simulink library "GenericTarget"  (R2020b)
settings: Solver=VariableStepAuto  StartTime=0.0  StopTime=10.0  RelTol=1e-3
undefined symbols (not defined in the file or in its folder): CheckUniqueParameterValue
(part 1 of 2)
settings Model: Creator=damerius  LastModifiedBy=damerius

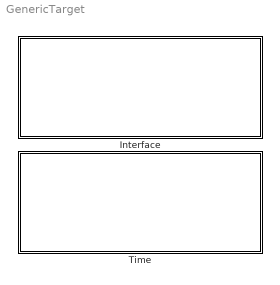
== system GenericTarget ==
  Interface : Subsystem
  Time : Subsystem

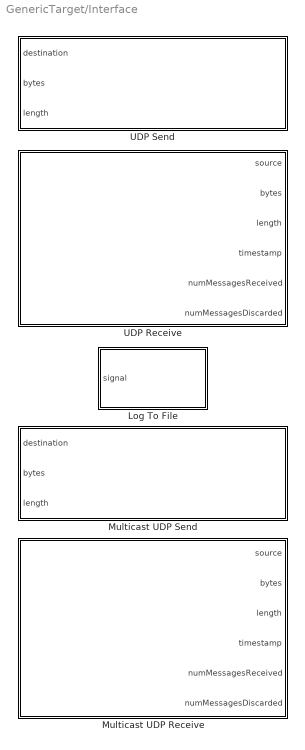
== system GenericTarget/Interface ==
  Log To File : Subsystem  InitFcn=CheckUniqueParameterValue(gcs,gcb,'idLog');  mask{idLog=0, signalDimension=1, labelsLog='label'}
      mask prompts: idLog "Unique ID:"; signalDimension "Signal dimension:"; labelsLog "Signal names, seperated by comma in one string:"
      mask help:
      | Log a signal to a file. This block implements the signal logging functionality on the generic target. During simulation this block has no effect.
      |
      | Internally, the model time is used as timestamp.
      mask DialogControl DescGroupVar Prompt: Log To File - Generic Target
      mask Display:
      | % Get dimension of block
      | pos = get_param(gcb, 'Position');
      | width = pos(3) - pos(1);
      | height = pos(4) - pos(2);
      | 
      | % Set image to center of block
      | imgSize = 32;
      | image('write.svg', [width-imgSize,0.5*(height-imgSize),imgSize,imgSize]);
      | image('icon.svg', [0.5*(width-imgSize),0.5*(height-imgSize),imgSize,imgSize]);
      | 
      | % Show socket port
      | maskStr = get_param(gcb,'idLog');
      | strText = ['ID: ' maskStr];
      | text(0.5*width,0.5*(height-imgSize)-4,strText, 'hor','center','texmode','on');
  Multicast UDP Receive : Subsystem  InitFcn=CheckUniqueParameterValue(gcs,gcb,'interfacePortRX');  mask{interfacePortRX=25000, interfaceIP=[0,0,0,0], groupIP=[239,0,0,0], rxBufferSize=1024, SampleTime=-1, prioritySocket=6, priorityThread=31, ttl=1, maxNumMessages=1, bufferStrategy=Discard oldest message}
      mask prompts: interfacePortRX "Local port:"; interfaceIP "Interface ([0,0,0,0] for default interface):"; groupIP "Group address:"; rxBufferSize "Receive buffer size:"; SampleTime "Sample time (-1 for inherited):"; prioritySocket "Socket priority (0 ... 6, default is 6):"; priorityThread "Receiver thread priority (0 ... 99, default is 31):"; ttl "Time-to-live value associated with multicast traffic for this socket (default is 1)"; maxNumMessages "Maximum number of messages in buffer (default is 1):"; bufferStrategy "Buffer strategy (if buffer is full):"
      mask help:
      | Receive UDP messages from a multicast group. This block implements the UDP multicast receiver functionality on the generic target. If the toolbox was built with the host implementation, then this block behaves similar to the one on the target. Otherwise this block has no effect during simulations.<br><br>
      |
      | <b>source</b><br>A 5-by-M uint16 vector denoting the source address, where M denotes the number of messages in the buffer. The first four values in a column indicate the source IPv4 address (LSB) and the fifth value in a column indicates the source port.<br><br>
      |
      | <b>bytes</b><br>An N-by-M matrix containing the messages that have been received, where N indicates the buffer size for a single message and M denotes the number of messages in the buffer.<br><br>
      |
      | <b>length</b><br>An M-by-1 vector indicating the actual length of the corresponding message.<br><br>
      |
      | <b>timestamp</b><br>An M-by-1 vector indicating the timestamp in seconds (model time) when the corresponding message has been received.<br><br>
      |
      | <b>numMessagesReceived</b><br>The number of messages that have been received.<br><br>
      |
      | <b>numMessagesDiscarded</b><br>The number of messages that have been discarded.
      mask TypeOptions bufferStrategy: Discard oldest message | Discard received message
      mask DialogControl DescGroupVar Prompt: Multicast UDP Receive - Generic Target
      mask DialogControl Container4 Prompt: Parameters
      mask DialogControl Container7 Prompt: Advanced
      mask DialogControl Container6 Prompt: Buffering
      mask Display:
      | % Get dimension of block
      | pos = get_param(gcb, 'Position');
      | width = pos(3) - pos(1);
      | height = pos(4) - pos(2);
      | 
      | % Set image to center of block
      | imgSize = 32;
      | image('rx.svg', [0,0.5*(height-imgSize),imgSize,imgSize]);
      | image('icon.svg', [0.5*(width-imgSize),0.5*(height-imgSize),imgSize,imgSize]);
      | 
      | % Show socket port
      | maskStr = get_param(gcb,'interfacePortRX');
      | strText = ['Port: ' maskStr];
      | text(0.5*width,0.5*(height-imgSize)-4,strText, 'hor','center','texmode','on');
      | 
      | % Show group ip
      | maskStr = get_param(gcb,'groupIP');
      | maskStr = strrep(maskStr,'[','');
      | maskStr = strrep(maskStr,']','');
      | maskStr = strrep(maskStr,',','.');
      | text(0.5*width,0.5*(height+imgSize)+6,maskStr, 'hor','center','texmode','on');
  Multicast UDP Send : Subsystem  mask{interfacePort=25000, groupIP=[239,0,0,0], interfaceIP=[0,0,0,0], SampleTime=-1, prioritySocket=6, priorityThread=31, ttl=1}
      mask prompts: interfacePort "Local port:"; groupIP "Group address:"; interfaceIP "Interface ([0,0,0,0] for default interface):"; SampleTime "Sample time (-1 for inherited):"; prioritySocket "Socket priority (0 ... 6, default is 6):"; priorityThread "Receiver thread priority (0 ... 99, default is 31):"; ttl "Time-to-live value associated with multicast traffic for this socket (default is 1):"
      mask help:
      | Send a UDP message to a specified destination. This block implements the UDP multicast transmission functionality on the generic target. If the toolbox was built with the host implementation, then this block behaves similar to the one on the target. Otherwise this block has no effect during simulations.<br><br>
      |
      | <b>destination</b><br>A 5-by-1 uint16 vector denoting the destination address, where the first four values indicate the destination IPv4 address (LSByte) and the fifth value indicates the destination port.<br><br>
      |
      | <b>bytes</b><br>The message that should be transmitted.<br><br>
      |
      | <b>length</b><br>The number of bytes that should be transmitted.
      mask DialogControl DescGroupVar Prompt: Multicast UDP Send - Generic Target
      mask DialogControl Container4 Prompt: Parameters
      mask DialogControl Container5 Prompt: Advanced
      mask Display:
      | % Get dimension of block
      | pos = get_param(gcb, 'Position');
      | width = pos(3) - pos(1);
      | height = pos(4) - pos(2);
      | 
      | % Set image to center of block
      | imgSize = 32;
      | image('tx.svg', [width-imgSize,0.5*(height-imgSize),imgSize,imgSize]);
      | image('icon.svg', [0.5*(width-imgSize),0.5*(height-imgSize),imgSize,imgSize]);
      | 
      | % Show socket port
      | maskStr = get_param(gcb,'interfacePort');
      | strText = ['Port: ' maskStr];
      | text(0.5*width,0.5*(height-imgSize)-4,strText, 'hor','center','texmode','on');
      | 
      | % Show group ip
      | maskStr = get_param(gcb,'groupIP');
      | maskStr = strrep(maskStr,'[','');
      | maskStr = strrep(maskStr,']','');
      | maskStr = strrep(maskStr,',','.');
      | text(0.5*width,0.5*(height+imgSize)+6,maskStr, 'hor','center','texmode','on');
  UDP Receive : Subsystem  InitFcn=CheckUniqueParameterValue(gcs,gcb,'interfacePortRX');  mask{interfacePortRX=25000, interfaceIP=[0,0,0,0], rxBufferSize=1024, SampleTime=-1, prioritySocket=6, priorityThread=31, maxNumMessages=1, bufferStrategy=Discard oldest message}
      mask prompts: interfacePortRX "Local port:"; interfaceIP "Interface ([0,0,0,0] for default interface):"; rxBufferSize "Receive buffer size:"; SampleTime "Sample time (-1 for inherited):"; prioritySocket "Socket priority (0 ... 6, default is 6):"; priorityThread "Receiver thread priority (0 ... 99, default is 31):"; maxNumMessages "Maximum number of messages in buffer (default is 1):"; bufferStrategy "Buffer strategy (if buffer is full):"
      mask help:
      | Receive UDP messages at the specified port. This block implements the UDP receiver functionality on the generic target. If the toolbox was built with the host implementation, then this block behaves similar to the one on the target. Otherwise this block has no effect during simulations.<br><br>
      |
      | <b>source</b><br>A 5-by-M uint16 vector denoting the source address, where M denotes the number of messages in the buffer. The first four values in a column indicate the source IPv4 address (LSB) and the fifth value in a column indicates the source port.<br><br>
      |
      | <b>bytes</b><br>An N-by-M matrix containing the messages that have been received, where N indicates the buffer size for a single message and M denotes the number of messages in the buffer.<br><br>
      |
      | <b>length</b><br>An M-by-1 vector indicating the actual length of the corresponding message.<br><br>
      |
      | <b>timestamp</b><br>An M-by-1 vector indicating the timestamp in seconds (model time) when the corresponding message has been received.<br><br>
      |
      | <b>numMessagesReceived</b><br>The number of messages that have been received.<br><br>
      |
      | <b>numMessagesDiscarded</b><br>The number of messages that have been discarded.
      mask TypeOptions bufferStrategy: Discard oldest message | Discard received message
      mask DialogControl DescGroupVar Prompt: UDP Receive - Generic Target
      mask DialogControl Container4 Prompt: Parameters
      mask DialogControl Container5 Prompt: Advanced
      mask DialogControl Container8 Prompt: Buffering
      mask Display:
      | % Get dimension of block
      | pos = get_param(gcb, 'Position');
      | width = pos(3) - pos(1);
      | height = pos(4) - pos(2);
      | 
      | % Set image to center of block
      | imgSize = 32;
      | image('rx.svg', [0,0.5*(height-imgSize),imgSize,imgSize]);
      | image('icon.svg', [0.5*(width-imgSize),0.5*(height-imgSize),imgSize,imgSize]);
      | 
      | % Show socket port
      | maskStr = get_param(gcb,'interfacePortRX');
      | strText = ['Port: ' maskStr];
      | text(0.5*width,0.5*(height-imgSize)-4,strText, 'hor','center','texmode','on');
  UDP Send : Subsystem  mask{interfacePort=25000, interfaceIP=[0,0,0,0], SampleTime=-1, prioritySocket=6, priorityThread=31}
      mask prompts: interfacePort "Local port:"; interfaceIP "Interface ([0,0,0,0] for default interface):"; SampleTime "Sample time (-1 for inherited):"; prioritySocket "Socket priority (0 ... 6, default is 6):"; priorityThread "Receiver thread priority (0 ... 99, default is 31):"
      mask help:
      | Send a UDP message to a specified destination. This block implements the UDP transmission functionality on the generic target. If the toolbox was built with the host implementation, then this block behaves similar to the one on the target. Otherwise this block has no effect during simulations.<br><br>
      |
      | <b>destination</b><br>A 5-by-1 uint16 vector denoting the destination address, where the first four values indicate the destination IPv4 address (LSByte) and the fifth value indicates the destination port.<br><br>
      |
      | <b>bytes</b><br>The message that should be transmitted.<br><br>
      |
      | <b>length</b><br>The number of bytes that should be transmitted.
      mask DialogControl DescGroupVar Prompt: UDP Send - Generic Target
      mask DialogControl Container12 Prompt: Parameters
      mask DialogControl Container13 Prompt: Advanced
      mask Display:
      | % Get dimension of block
      | pos = get_param(gcb, 'Position');
      | width = pos(3) - pos(1);
      | height = pos(4) - pos(2);
      | 
      | % Set image to center of block
      | imgSize = 32;
      | image('tx.svg', [width-imgSize,0.5*(height-imgSize),imgSize,imgSize]);
      | image('icon.svg', [0.5*(width-imgSize),0.5*(height-imgSize),imgSize,imgSize]);
      | 
      | % Show socket port
      | maskStr = get_param(gcb,'interfacePort');
      | strText = ['Port: ' maskStr];
      | text(0.5*width,0.5*(height-imgSize)-4,strText, 'hor','center','texmode','on');

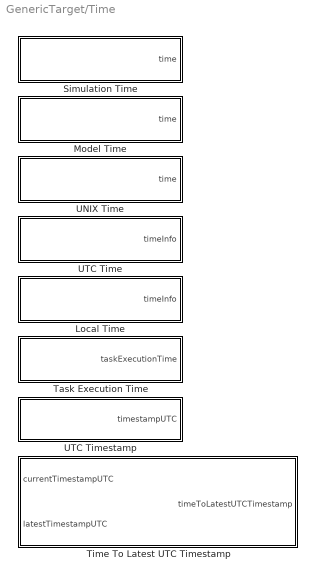
== system GenericTarget/Time ==
  Local Time : Subsystem  mask{SampleTime=-1}
      mask prompts: SampleTime "Sample time (-1 for inherited):"
      mask help:
      | Get the current local time of the target. If the toolbox was not built with the host implementation, then this block has no effect during simulations. If, however, the toolbox was built with the host implementation, then this blocks returns the current local time. The behaviour is different to that one on the target. During simulation each of these blocks returns the local time separately. However, on the target the local time is determined only once per base sampletime.<br><br>
      |
      | <b>nanoseconds</b><br>Nanoseconds after the second [0, 999999999].<br><br>
      |
      | <b>second</b><br>Seconds after the minute [0, 60] (60 to allow leap second).<br><br>
      |
      | <b>minute</b><br>Minutes after the hour [0, 59].<br><br>
      |
      | <b>hour</b><br>Hours since midnight [0, 23].<br><br>
      |
      | <b>mday</b><br>Day of the month [1, 31].<br><br>
      |
      | <b>mon</b><br>Month since January [0, 11].<br><br>
      |
      | <b>year</b><br>Years since 1900.<br><br>
      |
      | <b>wday</b><br>Days since Sunday [0, 6].<br><br>
      |
      | <b>yday</b><br>Days since January 1 [0, 365].<br><br>
      |
      | <b>isdst</b><br>Daylight Saving Time flag. The value is positive if DST is in effect, zero if not and negative if no information is available.
      mask DialogControl DescGroupVar Prompt: Local Time - Generic Target
      mask Display:
      | % Get dimension of block
      | pos = get_param(gcb, 'Position');
      | width = pos(3) - pos(1);
      | height = pos(4) - pos(2);
      | 
      | % Set image to center of block
      | imgSize = 32;
      | image('time.svg', [0.5*(height-imgSize),0.5*(height-imgSize),imgSize,imgSize]);
      | image('icon.svg', [0.5*(width-imgSize),0.5*(height-imgSize),imgSize,imgSize]);
      | 
      | % Set text
      | text(2,2,'Local','horizontalAlignment','left','verticalAlignment','bottom','texmode','on');
  Model Time : Subsystem  mask{SampleTime=-1}
      mask prompts: SampleTime "Sample time (-1 for inherited):"
      mask help:
      | Get the current execution time of the model. If the toolbox was not built with the host implementation, then this block has no effect during simulations. If, however, the toolbox was built with the host implementation, then this blocks returns the measured time to the simulation start. The behaviour is different to that one on the target. During simulation each of these blocks measures the model time separately. However, on the target the model time is measured only once per base sampletime.<br><br>
      |
      | <b>time</b><br>The execution time of the model in seconds.
      mask DialogControl DescGroupVar Prompt: Model Time - Generic Target
      mask Display:
      | % Get dimension of block
      | pos = get_param(gcb, 'Position');
      | width = pos(3) - pos(1);
      | height = pos(4) - pos(2);
      | 
      | % Set image to center of block
      | imgSize = 32;
      | image('time.svg', [0.5*(height-imgSize),0.5*(height-imgSize),imgSize,imgSize]);
      | image('icon.svg', [0.5*(width-imgSize),0.5*(height-imgSize),imgSize,imgSize]);
      | 
      | % Set text
      | text(2,2,'Model','horizontalAlignment','left','verticalAlignment','bottom','texmode','on');
  Simulation Time : Subsystem  mask{SampleTime=-1}
      mask prompts: SampleTime "Sample time (-1 for inherited):"
      mask help:
      | Get the current simulation time of the model. During simulation this block has no effect.<br><br>
      |
      | <b>time</b><br>The simulation time of the model in seconds, that is the number of ticks from of the base rate times the base sample time.
      mask DialogControl DescGroupVar Prompt: Simulation Time - Generic Target
      mask Display:
      | % Get dimension of block
      | pos = get_param(gcb, 'Position');
      | width = pos(3) - pos(1);
      | height = pos(4) - pos(2);
      | 
      | % Set image to center of block
      | imgSize = 32;
      | image('time.svg', [0.5*(height-imgSize),0.5*(height-imgSize),imgSize,imgSize]);
      | image('icon.svg', [0.5*(width-imgSize),0.5*(height-imgSize),imgSize,imgSize]);
      | 
      | % Set text
      | text(2,2,'Simulation','horizontalAlignment','left','verticalAlignment','bottom','texmode','on');
  Task Execution Time : Subsystem  mask{SampleTime=0.001}
      mask prompts: SampleTime "Sample time (<b>must be explicitly specified</b>):"
      mask help: Get the latest task execution time in seconds for the task running at the specified sampletime. During simulation this block has no effect.
      mask DialogControl DescGroupVar Prompt: Task Execution Time - Generic Target
      mask Display:
      | % Get dimension of block
      | pos = get_param(gcb, 'Position');
      | width = pos(3) - pos(1);
      | height = pos(4) - pos(2);
      | 
      | % Set image to center of block
      | imgSize = 32;
      | image('time.svg', [0.5*(height-imgSize),0.5*(height-imgSize),imgSize,imgSize]);
      | image('icon.svg', [0.5*(width-imgSize),0.5*(height-imgSize),imgSize,imgSize]);
      | 
      | % Set text
      | text(2,2,'TET','horizontalAlignment','left','verticalAlignment','bottom','texmode','on');
  Time To Latest UTC Timestamp : Subsystem
      mask help:
      | This block calculates the time difference (seconds) to the latest UTC timestamp. The block only uses standard simulink blocks.<br><br>
      | The basic behaviour is as follows:<br>
      | <b>output</b> = <b>current</b> - <b>latest</b>
      mask DialogControl DescGroupVar Prompt: Time To Latest UTC Timestamp
      mask Display:
      | % Get dimension of block
      | pos = get_param(gcb, 'Position');
      | width = pos(3) - pos(1);
      | height = pos(4) - pos(2);
      | 
      | % Set image to center of block
      | imgSize = 32;
      | image('icon.svg', [0.5*(width-imgSize),0.5*(height-imgSize),imgSize,imgSize]);
  UNIX Time : Subsystem  mask{SampleTime=-1}
      mask prompts: SampleTime "Sample time (-1 for inherited):"
      mask help:
      | Get the current UNIX time. If the toolbox was not built with the host implementation, then this block has no effect during simulations. If, however, the toolbox was built with the host implementation, then this blocks returns the current UNIX time. The behaviour is different to that one on the target. During simulation each of these blocks returns the UNIX time separately. However, on the target the UNIX time is determined only once per base sampletime.<br><br>
      |
      | <b>time</b><br>The UNIX time in seconds. The resolution is one millisecond.
      mask DialogControl DescGroupVar Prompt: UNIX Time - Generic Target
      mask Display:
      | % Get dimension of block
      | pos = get_param(gcb, 'Position');
      | width = pos(3) - pos(1);
      | height = pos(4) - pos(2);
      | 
      | % Set image to center of block
      | imgSize = 32;
      | image('time.svg', [0.5*(height-imgSize),0.5*(height-imgSize),imgSize,imgSize]);
      | image('icon.svg', [0.5*(width-imgSize),0.5*(height-imgSize),imgSize,imgSize]);
      | 
      | % Set text
      | text(2,2,'UNIX','horizontalAlignment','left','verticalAlignment','bottom','texmode','on');
  UTC Time : Subsystem  mask{SampleTime=-1}
      mask prompts: SampleTime "Sample time (-1 for inherited):"
      mask help:
      | Get the current UTC time of the target. If the toolbox was not built with the host implementation, then this block has no effect during simulations. If, however, the toolbox was built with the host implementation, then this blocks returns the current UTC time. The behaviour is different to that one on the target. During simulation each of these blocks returns the UTC time separately. However, on the target the UTC time is determined only once per base sampletime.<br><br>
      |
      | <b>nanoseconds</b><br>Nanoseconds after the second [0, 999999999].<br><br>
      |
      | <b>second</b><br>Seconds after the minute [0, 60] (60 to allow leap second).<br><br>
      |
      | <b>minute</b><br>Minutes after the hour [0, 59].<br><br>
      |
      | <b>hour</b><br>Hours since midnight [0, 23].<br><br>
      |
      | <b>mday</b><br>Day of the month [1, 31].<br><br>
      |
      | <b>mon</b><br>Month since January [0, 11].<br><br>
      |
      | <b>year</b><br>Years since 1900.<br><br>
      |
      | <b>wday</b><br>Days since Sunday [0, 6].<br><br>
      |
      | <b>yday</b><br>Days since January 1 [0, 365].<br><br>
      |
      | <b>isdst</b><br>Daylight Saving Time flag. The value is positive if DST is in effect, zero if not and negative if no information is available.
      mask DialogControl DescGroupVar Prompt: UTC Time - Generic Target
      mask Display:
      | % Get dimension of block
      | pos = get_param(gcb, 'Position');
      | width = pos(3) - pos(1);
      | height = pos(4) - pos(2);
      | 
      | % Set image to center of block
      | imgSize = 32;
      | image('time.svg', [0.5*(height-imgSize),0.5*(height-imgSize),imgSize,imgSize]);
      | image('icon.svg', [0.5*(width-imgSize),0.5*(height-imgSize),imgSize,imgSize]);
      | 
      | % Set text
      | text(2,2,'UTC','horizontalAlignment','left','verticalAlignment','bottom','texmode','on');
  UTC Timestamp : Subsystem  mask{SampleTime=-1}
      mask prompts: SampleTime "Sample time (-1 for inherited):"
      mask help:
      | Get the current UTC timestamp. If the toolbox was not built with the host implementation, then this block has no effect during simulations. If, however, the toolbox was built with the host implementation, then this blocks returns the current UTC timestamp. The behaviour is different to that one on the target. During simulation each of these blocks returns the UTC timestamp separately. However, on the target the UTC timestamp is determined only once per base sampletime.<br><br>
      |
      | <b>timestampUTC</b><br>UTC second of the day.
      mask DialogControl DescGroupVar Prompt: UTC Timestamp - Generic Target
      mask Display:
      | % Get dimension of block
      | pos = get_param(gcb, 'Position');
      | width = pos(3) - pos(1);
      | height = pos(4) - pos(2);
      | 
      | % Set image to center of block
      | imgSize = 32;
      | image('time.svg', [0.5*(height-imgSize),0.5*(height-imgSize),imgSize,imgSize]);
      | image('icon.svg', [0.5*(width-imgSize),0.5*(height-imgSize),imgSize,imgSize]);
      | 
      | % Set text
      | text(2,2,'UTC','horizontalAlignment','left','verticalAlignment','bottom','texmode','on');

== system GenericTarget/Interface/Log To File ==
  signal : Inport  OutDataTypeStr=double  PortDimensions=signalDimension
  SFunctionDriverSignalLog : S-Function  FunctionName=SFunctionDriverSignalLog  Parameters=SParameter1, SParameter2, SParameter3, SParameter4, SampleTime  SFunctionDeploymentMode=off  EnableBusSupport=off  mask(Legacy Function){SFunctionSpec=void OutputDriverSignalLog(uint32 p1, double u1[p2], uint32 p2), SParameter1=uint32(reshape(idLog, [1 1])), SParameter2=uint32(reshape(signalDimension, [1 1])), SParameter3=uint8(labelsLog), SParameter4=uint32(length(labelsLog)), SampleTime=-1, ShowSpec=on}
      mask prompts: SParameter1 "P1:"; SParameter2 "P2:"; SParameter3 "P3:"; SParameter4 "P4:"; SampleTime "Sample time (-1 for inherited):"; ShowSpec "Display function specification"
      mask help:
      | This block allows you to call the legacy functions specified by the following Legacy Code Tool definition:
      | def.SFunctionName = 'SFunctionDriverSignalLog';
      | def.OutputFcnSpec = 'void OutputDriverSignalLog(uint32 p1, double u1[p2], uint32 p2)';
      | def.StartFcnSpec = 'void CreateDriverSignalLog(uint32 p1, uint32 p2, uint8 p3[], uint32 p4)';
      | def.TerminateFcnSpec = 'void DeleteDriverSignalLog()';
      | def.HeaderFiles = {'DriverSignalLog.h'};
      | def.SourceFiles = {'DriverSignalLog.cpp'};
      | def.SampleTime = 'parameterized';
      | def.Options.useTlcWithAccel = false;
      mask Help: <p>This block was generated automatically by the Legacy Code Tool. For detailed help on this tool, call<a href="matlab:legacy_code('help')"> legacy_code('help')</a>.</p>
      mask Callback ShowSpec:
      | if strcmp(get_param(gcbh, 'ShowSpec'), 'on')
      |   set_param(gcbh, 'MaskDisplay', sprintf('fprintf(''%s'');', get_param(gcbh, 'SFunctionSpec')));
      | else
      |   set_param(gcbh, 'MaskDisplay', sprintf('fprintf(''%s'');', get_param(gcbh, 'FunctionName')));
      | end
      mask Display: fprintf('void OutputDriverSignalLog(uint32 p1, double u1[p2], uint32 p2)');
  wires:
  signal/1 -> SFunctionDriverSignalLog/1

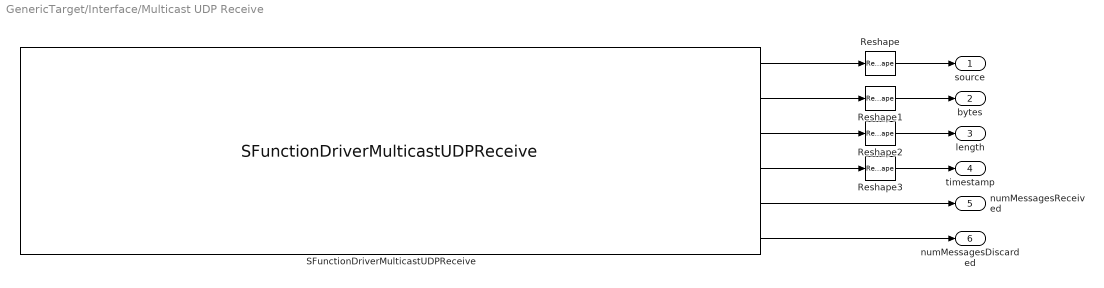
== system GenericTarget/Interface/Multicast UDP Receive ==
  Reshape : Reshape  OutputDimensionality=Customize  OutputDimensions=[5,maxNumMessages]
  Reshape1 : Reshape  OutputDimensionality=Customize  OutputDimensions=[rxBufferSize,maxNumMessages]
  Reshape2 : Reshape  OutputDimensionality=Customize  OutputDimensions=[maxNumMessages,1]
  Reshape3 : Reshape  OutputDimensionality=Customize  OutputDimensions=[maxNumMessages,1]
  SFunctionDriverMulticastUDPReceive : S-Function  FunctionName=SFunctionDriverMulticastUDPReceive  Parameters=SParameter1, SParameter2, SParameter3, SParameter4, SParameter5, SParameter6, SParameter7, SParameter8, SParameter9, SampleTime  SFunctionDeploymentMode=off  EnableBusSupport=off  mask(Legacy Function){SFunctionSpec=void OutputDriverMulticastUDPReceive(uint16 p1, uint32 p4, uint32 p8, uint16 y1[5*p8], uint8 y2[p4*p8], uint32 y3[p8], double y4[p8], uint32 y5[1], uint32 y6[1]), SParameter1=uint16(reshape(interfacePortRX, [1,1])), SParameter2=uint8(reshape(interfaceIP, [4,1])), SParameter3=uint8(reshape(groupIP, [4,1])), SParameter4=uint32(reshape(rxBufferSize, [1,1])), SParameter5=int32(reshape(prioritySocket, [1,1])), SParameter6=int32(reshape(priorityThread, [1,1])), SParameter7=uint8(reshape(ttl, [1,1])), SParameter8=uint32(reshape(maxNumMessages, [1,1])), SParameter9=uint32(reshape(bufferStrategy, [1,1]) - 1), SampleTime=SampleTime, ShowSpec=on}
      mask prompts: SParameter1 "P1:"; SParameter2 "P2:"; SParameter3 "P3:"; SParameter4 "P4:"; SParameter5 "P5:"; SParameter6 "P6:"; SParameter7 "P7:"; SParameter8 "P8:"; SParameter9 "P9:"; SampleTime "Sample time (-1 for inherited):"; ShowSpec "Display function specification"
      mask help:
      | This block allows you to call the legacy functions specified by the following Legacy Code Tool definition:
      | def.SFunctionName = 'SFunctionDriverMulticastUDPReceive';
      | def.OutputFcnSpec = 'void OutputDriverMulticastUDPReceive(uint16 p1, uint32 p4, uint32 p8, uint16 y1[5*p8], uint8 y2[p4*p8], uint32 y3[p8], double y4[p8], uint32 y5[1], uint32 y6[1])';
      | def.StartFcnSpec = 'void CreateDriverMulticastUDPReceive(uint16 p1, uint8 p2[4], uint8 p3[4], uint32 p4, int32 p5, int32 p6, uint8 p7, uint32 p8, uint32 p9)';
      | def.TerminateFcnSpec = 'void DeleteDriverMulticastUDPReceive()';
      | def.HeaderFiles = {'DriverMulticastUDPReceive.h'};
      | def.SourceFiles = {'DriverMulticastUDPReceive.cpp'};
      | def.SampleTime = 'parameterized';
      | def.Options.useTlcWithAccel = false;
      mask Help: <p>This block was generated automatically by the Legacy Code Tool. For detailed help on this tool, call<a href="matlab:legacy_code('help')"> legacy_code('help')</a>.</p>
      mask Callback ShowSpec:
      | if strcmp(get_param(gcbh, 'ShowSpec'), 'on')
      |   set_param(gcbh, 'MaskDisplay', sprintf('fprintf(''%s'');', get_param(gcbh, 'SFunctionSpec')));
      | else
      |   set_param(gcbh, 'MaskDisplay', sprintf('fprintf(''%s'');', get_param(gcbh, 'FunctionName')));
      | end
      mask Display: fprintf('void OutputDriverMulticastUDPReceive(uint16 p1, uint32 p4, uint32 p8, uint16 y1[5*p8], uint8 y2[p4*p8], uint32 y3[p8], double y4[p8], uint32 y5[1], uint32 y6[1])');
  source : Outport  OutDataTypeStr=uint16  PortDimensions=[5,maxNumMessages]  VectorParamsAs1DForOutWhenUnconnected=off
  bytes : Outport  Port=2  OutDataTypeStr=uint8  PortDimensions=[rxBufferSize,maxNumMessages]  VectorParamsAs1DForOutWhenUnconnected=off
  length : Outport  Port=3  OutDataTypeStr=uint32  PortDimensions=[maxNumMessages,1]  VectorParamsAs1DForOutWhenUnconnected=off
  timestamp : Outport  Port=4  OutDataTypeStr=double  Unit=s  PortDimensions=[maxNumMessages,1]  VectorParamsAs1DForOutWhenUnconnected=off
  numMessagesReceived : Outport  Port=5  OutDataTypeStr=uint32  PortDimensions=1  VectorParamsAs1DForOutWhenUnconnected=off
  numMessagesDiscarded : Outport  Port=6  OutDataTypeStr=uint32  PortDimensions=1  VectorParamsAs1DForOutWhenUnconnected=off
  wires:
  SFunctionDriverMulticastUDPReceive/4 -> Reshape3/1
  SFunctionDriverMulticastUDPReceive/3 -> Reshape2/1
  SFunctionDriverMulticastUDPReceive/2 -> Reshape1/1
  SFunctionDriverMulticastUDPReceive/1 -> Reshape/1
  Reshape/1 -> source/1
  Reshape1/1 -> bytes/1
  Reshape2/1 -> length/1
  Reshape3/1 -> timestamp/1
  SFunctionDriverMulticastUDPReceive/5 -> numMessagesReceived/1
  SFunctionDriverMulticastUDPReceive/6 -> numMessagesDiscarded/1

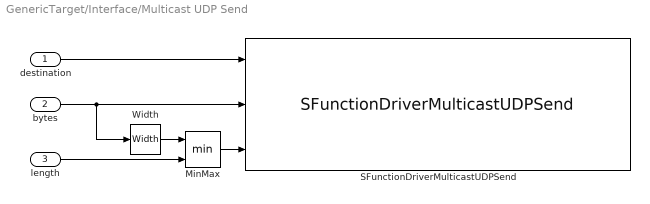
== system GenericTarget/Interface/Multicast UDP Send ==
  destination : Inport  OutDataTypeStr=uint16  PortDimensions=5
  bytes : Inport  Port=2  OutDataTypeStr=uint8
  length : Inport  Port=3  OutDataTypeStr=uint32  PortDimensions=1
  MinMax : MinMax  Inputs=2  OutDataTypeStr=uint32
  SFunctionDriverMulticastUDPSend : S-Function  FunctionName=SFunctionDriverMulticastUDPSend  Parameters=SParameter1, SParameter2, SParameter3, SParameter4, SParameter5, SParameter6, SampleTime  SFunctionDeploymentMode=off  EnableBusSupport=off  mask(Legacy Function){SFunctionSpec=void OutputDriverMulticastUDPSend(uint16 p1, uint16 u1[5], uint8 u2[], uint32 u3), SParameter1=uint16(reshape(interfacePort, [1,1])), SParameter2=uint8(reshape(interfaceIP, [4,1])), SParameter3=uint8(reshape(groupIP, [4,1])), SParameter4=int32(reshape(prioritySocket, [1,1])), SParameter5=int32(reshape(priorityThread, [1,1])), SParameter6=uint8(reshape(ttl, [1,1])), SampleTime=SampleTime, ShowSpec=on}
      mask prompts: SParameter1 "P1:"; SParameter2 "P2:"; SParameter3 "P3:"; SParameter4 "P4:"; SParameter5 "P5:"; SParameter6 "P6:"; SampleTime "Sample time (-1 for inherited):"; ShowSpec "Display function specification"
      mask help:
      | This block allows you to call the legacy functions specified by the following Legacy Code Tool definition:
      | def.SFunctionName = 'SFunctionDriverMulticastUDPSend';
      | def.OutputFcnSpec = 'void OutputDriverMulticastUDPSend(uint16 p1, uint16 u1[5], uint8 u2[], uint32 u3)';
      | def.StartFcnSpec = 'void CreateDriverMulticastUDPSend(uint16 p1, uint8 p2[4], uint8 p3[4], int32 p4, int32 p5, uint8 p6)';
      | def.TerminateFcnSpec = 'void DeleteDriverMulticastUDPSend()';
      | def.HeaderFiles = {'DriverMulticastUDPSend.h'};
      | def.SourceFiles = {'DriverMulticastUDPSend.cpp', 'HostImplementation.cpp'};
      | def.HostLibFiles = {'C:\Env\MSYS2\mingw64\x86_64-w64-mingw32\lib\libws2_32.a'};
      | def.SampleTime = 'parameterized';
      | def.Options.useTlcWithAccel = false;
      mask Help: <p>This block was generated automatically by the Legacy Code Tool. For detailed help on this tool, call<a href="matlab:legacy_code('help')"> legacy_code('help')</a>.</p>
      mask Callback ShowSpec:
      | if strcmp(get_param(gcbh, 'ShowSpec'), 'on')
      |   set_param(gcbh, 'MaskDisplay', sprintf('fprintf(''%s'');', get_param(gcbh, 'SFunctionSpec')));
      | else
      |   set_param(gcbh, 'MaskDisplay', sprintf('fprintf(''%s'');', get_param(gcbh, 'FunctionName')));
      | end
      mask Display: fprintf('void OutputDriverMulticastUDPSend(uint16 p1, uint16 u1[5], uint8 u2[], uint32 u3)');
  Width : Width  DataType=uint32
  wires:
  bytes/1 -> Width/1, SFunctionDriverMulticastUDPSend/2
  length/1 -> MinMax/2
  Width/1 -> MinMax/1
  MinMax/1 -> SFunctionDriverMulticastUDPSend/3
  destination/1 -> SFunctionDriverMulticastUDPSend/1

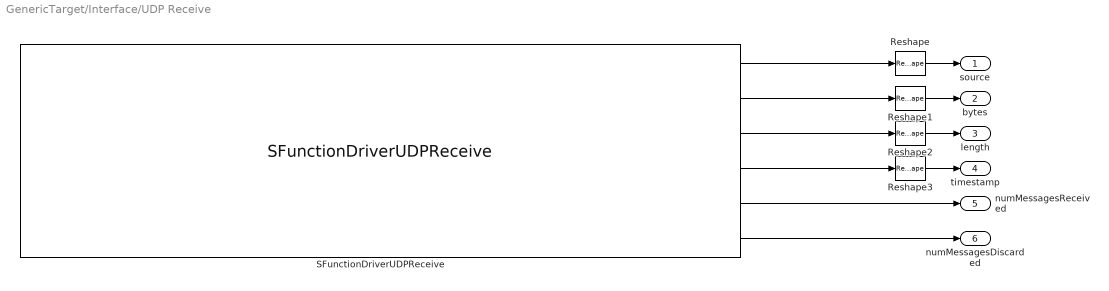
== system GenericTarget/Interface/UDP Receive ==
  Reshape : Reshape  OutputDimensionality=Customize  OutputDimensions=[5,maxNumMessages]
  Reshape1 : Reshape  OutputDimensionality=Customize  OutputDimensions=[rxBufferSize,maxNumMessages]
  Reshape2 : Reshape  OutputDimensionality=Customize  OutputDimensions=[maxNumMessages,1]
  Reshape3 : Reshape  OutputDimensionality=Customize  OutputDimensions=[maxNumMessages,1]
  SFunctionDriverUDPReceive : S-Function  FunctionName=SFunctionDriverUDPReceive  Parameters=SParameter1, SParameter2, SParameter3, SParameter4, SParameter5, SParameter6, SParameter7, SampleTime  SFunctionDeploymentMode=off  EnableBusSupport=off  mask(Legacy Function){SFunctionSpec=void OutputDriverUDPReceive(uint16 p1, uint32 p3, uint32 p6, uint16 y1[5*p6], uint8 y2[p3*p6], uint32 y3[p6], double y4[p6], uint32 y5[1], uint32 y6[1]), SParameter1=uint16(reshape(interfacePortRX, [1,1])), SParameter2=uint8(reshape(interfaceIP, [4,1])), SParameter3=uint32(reshape(rxBufferSize, [1,1])), SParameter4=int32(reshape(prioritySocket, [1,1])), SParameter5=int32(reshape(priorityThread, [1,1])), SParameter6=uint32(reshape(maxNumMessages, [1,1])), SParameter7=uint32(reshape(bufferStrategy, [1,1]) - 1), SampleTime=SampleTime, ShowSpec=on}
      mask prompts: SParameter1 "P1:"; SParameter2 "P2:"; SParameter3 "P3:"; SParameter4 "P4:"; SParameter5 "P5:"; SParameter6 "P6:"; SParameter7 "P7:"; SampleTime "Sample time (-1 for inherited):"; ShowSpec "Display function specification"
      mask help:
      | This block allows you to call the legacy functions specified by the following Legacy Code Tool definition:
      | def.SFunctionName = 'SFunctionDriverUDPReceive';
      | def.OutputFcnSpec = 'void OutputDriverUDPReceive(uint16 p1, uint32 p3, uint32 p6, uint16 y1[5*p6], uint8 y2[p3*p6], uint32 y3[p6], double y4[p6], uint32 y5[1], uint32 y6[1])';
      | def.StartFcnSpec = 'void CreateDriverUDPReceive(uint16 p1, uint8 p2[4], uint32 p3, int32 p4, int32 p5, uint32 p6, uint32 p7)';
      | def.TerminateFcnSpec = 'void DeleteDriverUDPReceive()';
      | def.HeaderFiles = {'DriverUDPReceive.h'};
      | def.SourceFiles = {'DriverUDPReceive.cpp'};
      | def.SampleTime = 'parameterized';
      | def.Options.useTlcWithAccel = false;
      mask Help: <p>This block was generated automatically by the Legacy Code Tool. For detailed help on this tool, call<a href="matlab:legacy_code('help')"> legacy_code('help')</a>.</p>
      mask Callback ShowSpec:
      | if strcmp(get_param(gcbh, 'ShowSpec'), 'on')
      |   set_param(gcbh, 'MaskDisplay', sprintf('fprintf(''%s'');', get_param(gcbh, 'SFunctionSpec')));
      | else
      |   set_param(gcbh, 'MaskDisplay', sprintf('fprintf(''%s'');', get_param(gcbh, 'FunctionName')));
      | end
      mask Display: fprintf('void OutputDriverUDPReceive(uint16 p1, uint32 p3, uint32 p6, uint16 y1[5*p6], uint8 y2[p3*p6], uint32 y3[p6], double y4[p6], uint32 y5[1], uint32 y6[1])');
  source : Outport  OutDataTypeStr=uint16  PortDimensions=[5,maxNumMessages]  VectorParamsAs1DForOutWhenUnconnected=off
  bytes : Outport  Port=2  OutDataTypeStr=uint8  PortDimensions=[rxBufferSize,maxNumMessages]  VectorParamsAs1DForOutWhenUnconnected=off
  length : Outport  Port=3  OutDataTypeStr=uint32  PortDimensions=[maxNumMessages,1]  VectorParamsAs1DForOutWhenUnconnected=off
  timestamp : Outport  Port=4  OutDataTypeStr=double  Unit=s  PortDimensions=[maxNumMessages,1]  VectorParamsAs1DForOutWhenUnconnected=off
  numMessagesReceived : Outport  Port=5  OutDataTypeStr=uint32  PortDimensions=1  VectorParamsAs1DForOutWhenUnconnected=off
  numMessagesDiscarded : Outport  Port=6  OutDataTypeStr=uint32  PortDimensions=1  VectorParamsAs1DForOutWhenUnconnected=off
  wires:
  SFunctionDriverUDPReceive/1 -> Reshape/1
  SFunctionDriverUDPReceive/2 -> Reshape1/1
  SFunctionDriverUDPReceive/3 -> Reshape2/1
  SFunctionDriverUDPReceive/4 -> Reshape3/1
  Reshape/1 -> source/1
  Reshape1/1 -> bytes/1
  Reshape2/1 -> length/1
  Reshape3/1 -> timestamp/1
  SFunctionDriverUDPReceive/5 -> numMessagesReceived/1
  SFunctionDriverUDPReceive/6 -> numMessagesDiscarded/1

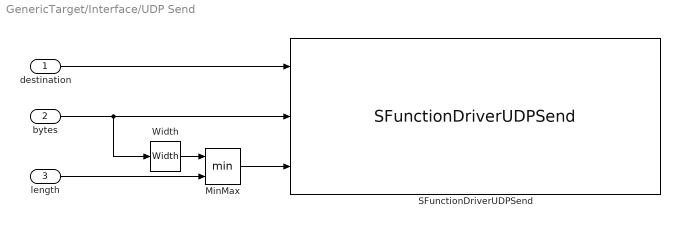
== system GenericTarget/Interface/UDP Send ==
  destination : Inport  OutDataTypeStr=uint16  PortDimensions=5
  bytes : Inport  Port=2  OutDataTypeStr=uint8
  length : Inport  Port=3  OutDataTypeStr=uint32  PortDimensions=1
  MinMax : MinMax  Inputs=2  OutDataTypeStr=uint32
  SFunctionDriverUDPSend : S-Function  FunctionName=SFunctionDriverUDPSend  Parameters=SParameter1, SParameter2, SParameter3, SParameter4, SampleTime  SFunctionDeploymentMode=off  EnableBusSupport=off  mask(Legacy Function){SFunctionSpec=void OutputDriverUDPSend(uint16 p1, uint16 u1[5], uint8 u2[], uint32 u3), SParameter1=uint16(reshape(interfacePort, [1,1])), SParameter2=uint8(reshape(interfaceIP, [4,1])), SParameter3=int32(reshape(prioritySocket, [1,1])), SParameter4=int32(reshape(priorityThread, [1,1])), SampleTime=SampleTime, ShowSpec=on}
      mask prompts: SParameter1 "P1:"; SParameter2 "P2:"; SParameter3 "P3:"; SParameter4 "P4:"; SampleTime "Sample time (-1 for inherited):"; ShowSpec "Display function specification"
      mask help:
      | This block allows you to call the legacy functions specified by the following Legacy Code Tool definition:
      | def.SFunctionName = 'SFunctionDriverUDPSend';
      | def.OutputFcnSpec = 'void OutputDriverUDPSend(uint16 p1, uint16 u1[5], uint8 u2[], uint32 u3)';
      | def.StartFcnSpec = 'void CreateDriverUDPSend(uint16 p1, uint8 p2[4], int32 p3, int32 p4)';
      | def.TerminateFcnSpec = 'void DeleteDriverUDPSend()';
      | def.HeaderFiles = {'DriverUDPSend.h'};
      | def.SourceFiles = {'DriverUDPSend.cpp', 'HostImplementation.cpp'};
      | def.SampleTime = 'parameterized';
      | def.Options.useTlcWithAccel = false;
      mask Help: <p>This block was generated automatically by the Legacy Code Tool. For detailed help on this tool, call<a href="matlab:legacy_code('help')"> legacy_code('help')</a>.</p>
      mask Callback ShowSpec:
      | if strcmp(get_param(gcbh, 'ShowSpec'), 'on')
      |   set_param(gcbh, 'MaskDisplay', sprintf('fprintf(''%s'');', get_param(gcbh, 'SFunctionSpec')));
      | else
      |   set_param(gcbh, 'MaskDisplay', sprintf('fprintf(''%s'');', get_param(gcbh, 'FunctionName')));
      | end
      mask Display: fprintf('void OutputDriverUDPSend(uint16 p1, uint16 u1[5], uint8 u2[], uint32 u3)');
  Width : Width  DataType=uint32
  wires:
  destination/1 -> SFunctionDriverUDPSend/1
  length/1 -> MinMax/2
  MinMax/1 -> SFunctionDriverUDPSend/3
  bytes/1 -> SFunctionDriverUDPSend/2, Width/1
  Width/1 -> MinMax/1

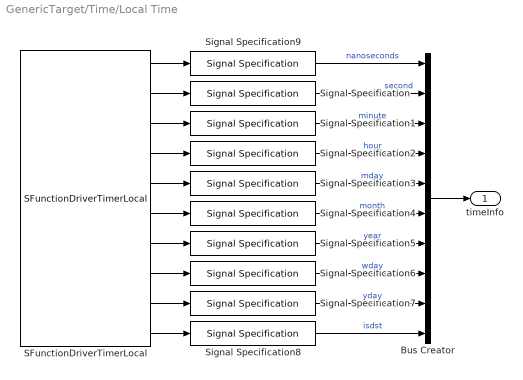
== system GenericTarget/Time/Local Time ==
  Bus Creator : BusCreator  Inputs=10
  SFunctionDriverTimerLocal : S-Function  FunctionName=SFunctionDriverTimerLocal  Parameters=SampleTime  SFunctionDeploymentMode=off  EnableBusSupport=off  mask(Legacy Function){SFunctionSpec=void OutputDriverTimerLocal(int32 y1[1], int32 y2[1], int32 y3[1], int32 y4[1], int32 y5[1], int32 y6[1], int32 y7[1], int32 y8[1], int32 y9[1], int32 y10[1]), SampleTime=SampleTime, ShowSpec=off}
      mask prompts: SampleTime "Sample time (-1 for inherited):"; ShowSpec "Display function specification"
      mask help:
      | This block allows you to call the legacy functions specified by the following Legacy Code Tool definition:
      | def.SFunctionName = 'SFunctionDriverTimerLocal';
      | def.OutputFcnSpec = 'void OutputDriverTimerLocal(int32 y1[1], int32 y2[1], int32 y3[1], int32 y4[1], int32 y5[1], int32 y6[1], int32 y7[1], int32 y8[1], int32 y9[1], int32 y10[1])';
      | def.StartFcnSpec = 'void CreateDriverTimerLocal()';
      | def.TerminateFcnSpec = 'void DeleteDriverTimerLocal()';
      | def.HeaderFiles = {'DriverTimerLocal.h'};
      | def.SourceFiles = {'DriverTimerLocal.cpp'};
      | def.SampleTime = 'parameterized';
      | def.Options.useTlcWithAccel = false;
      mask Help: <p>This block was generated automatically by the Legacy Code Tool. For detailed help on this tool, call<a href="matlab:legacy_code('help')"> legacy_code('help')</a>.</p>
      mask Callback ShowSpec:
      | if strcmp(get_param(gcbh, 'ShowSpec'), 'on')
      |   set_param(gcbh, 'MaskDisplay', sprintf('fprintf(''%s'');', get_param(gcbh, 'SFunctionSpec')));
      | else
      |   set_param(gcbh, 'MaskDisplay', sprintf('fprintf(''%s'');', get_param(gcbh, 'FunctionName')));
      | end
      mask Display: fprintf('SFunctionDriverTimerLocal');
  Signal Specification : SignalSpecification  OutDataTypeStr=int32  Unit=s  Dimensions=1
  Signal Specification1 : SignalSpecification  OutDataTypeStr=int32  Unit=min  Dimensions=1
  Signal Specification2 : SignalSpecification  OutDataTypeStr=int32  Unit=h  Dimensions=1
  Signal Specification3 : SignalSpecification  OutDataTypeStr=int32  Unit=d  Dimensions=1
  Signal Specification4 : SignalSpecification  OutDataTypeStr=int32  Dimensions=1
  Signal Specification5 : SignalSpecification  OutDataTypeStr=int32  Dimensions=1
  Signal Specification6 : SignalSpecification  OutDataTypeStr=int32  Unit=d  Dimensions=1
  Signal Specification7 : SignalSpecification  OutDataTypeStr=int32  Unit=d  Dimensions=1
  Signal Specification8 : SignalSpecification  OutDataTypeStr=int32  Dimensions=1
  Signal Specification9 : SignalSpecification  OutDataTypeStr=int32  Unit=ns  Dimensions=1
  timeInfo : Outport  VectorParamsAs1DForOutWhenUnconnected=off
  wires:
  Signal Specification/1 -> Bus Creator/2  "second"
  Signal Specification3/1 -> Bus Creator/5  "mday"
  Signal Specification4/1 -> Bus Creator/6  "month"
  Signal Specification1/1 -> Bus Creator/3  "minute"
  Signal Specification2/1 -> Bus Creator/4  "hour"
  Bus Creator/1 -> timeInfo/1
  Signal Specification5/1 -> Bus Creator/7  "year"
  Signal Specification6/1 -> Bus Creator/8  "wday"
  Signal Specification7/1 -> Bus Creator/9  "yday"
  Signal Specification8/1 -> Bus Creator/10  "isdst"
  Signal Specification9/1 -> Bus Creator/1  "nanoseconds"
  SFunctionDriverTimerLocal/1 -> Signal Specification9/1
  SFunctionDriverTimerLocal/2 -> Signal Specification/1
  SFunctionDriverTimerLocal/3 -> Signal Specification1/1
  SFunctionDriverTimerLocal/4 -> Signal Specification2/1
  SFunctionDriverTimerLocal/5 -> Signal Specification3/1
  SFunctionDriverTimerLocal/6 -> Signal Specification4/1
  SFunctionDriverTimerLocal/7 -> Signal Specification5/1
  SFunctionDriverTimerLocal/8 -> Signal Specification6/1
  SFunctionDriverTimerLocal/9 -> Signal Specification7/1
  SFunctionDriverTimerLocal/10 -> Signal Specification8/1

== system GenericTarget/Time/Model Time ==
  SFunctionDriverTimerModel : S-Function  FunctionName=SFunctionDriverTimerModel  Parameters=SampleTime  SFunctionDeploymentMode=off  EnableBusSupport=off  mask(Legacy Function){SFunctionSpec=void OutputDriverTimerModel(double y1[1]), SampleTime=SampleTime, ShowSpec=on}
      mask prompts: SampleTime "Sample time (-1 for inherited):"; ShowSpec "Display function specification"
      mask help:
      | This block allows you to call the legacy functions specified by the following Legacy Code Tool definition:
      | def.SFunctionName = 'SFunctionDriverTimerModel';
      | def.OutputFcnSpec = 'void OutputDriverTimerModel(double y1[1])';
      | def.StartFcnSpec = 'void CreateDriverTimerModel()';
      | def.TerminateFcnSpec = 'void DeleteDriverTimerModel()';
      | def.HeaderFiles = {'DriverTimerModel.h'};
      | def.SourceFiles = {'DriverTimerModel.cpp'};
      | def.SampleTime = 'parameterized';
      | def.Options.useTlcWithAccel = false;
      mask Help: <p>This block was generated automatically by the Legacy Code Tool. For detailed help on this tool, call<a href="matlab:legacy_code('help')"> legacy_code('help')</a>.</p>
      mask Callback ShowSpec:
      | if strcmp(get_param(gcbh, 'ShowSpec'), 'on')
      |   set_param(gcbh, 'MaskDisplay', sprintf('fprintf(''%s'');', get_param(gcbh, 'SFunctionSpec')));
      | else
      |   set_param(gcbh, 'MaskDisplay', sprintf('fprintf(''%s'');', get_param(gcbh, 'FunctionName')));
      | end
      mask Display: fprintf('void OutputDriverTimerModel(double y1[1])');
  time : Outport  OutDataTypeStr=double  Unit=s  PortDimensions=1  VectorParamsAs1DForOutWhenUnconnected=off
  wires:
  SFunctionDriverTimerModel/1 -> time/1

== system GenericTarget/Time/Simulation Time ==
  SFunctionDriverTimerSimulation : S-Function  FunctionName=SFunctionDriverTimerSimulation  Parameters=SampleTime  SFunctionDeploymentMode=off  EnableBusSupport=off  mask(Legacy Function){SFunctionSpec=void OutputDriverTimerSimulation(double y1[1]), SampleTime=SampleTime, ShowSpec=on}
      mask prompts: SampleTime "Sample time (-1 for inherited):"; ShowSpec "Display function specification"
      mask help:
      | This block allows you to call the legacy functions specified by the following Legacy Code Tool definition:
      | def.SFunctionName = 'SFunctionDriverTimerSimulation';
      | def.OutputFcnSpec = 'void OutputDriverTimerSimulation(double y1[1])';
      | def.StartFcnSpec = 'void CreateDriverTimerSimulation()';
      | def.TerminateFcnSpec = 'void DeleteDriverTimerSimulation()';
      | def.HeaderFiles = {'DriverTimerSimulation.h'};
      | def.SourceFiles = {'DriverTimerSimulation.cpp'};
      | def.SampleTime = 'parameterized';
      | def.Options.useTlcWithAccel = false;
      mask Help: <p>This block was generated automatically by the Legacy Code Tool. For detailed help on this tool, call<a href="matlab:legacy_code('help')"> legacy_code('help')</a>.</p>
      mask Callback ShowSpec:
      | if strcmp(get_param(gcbh, 'ShowSpec'), 'on')
      |   set_param(gcbh, 'MaskDisplay', sprintf('fprintf(''%s'');', get_param(gcbh, 'SFunctionSpec')));
      | else
      |   set_param(gcbh, 'MaskDisplay', sprintf('fprintf(''%s'');', get_param(gcbh, 'FunctionName')));
      | end
      mask Display: fprintf('void OutputDriverTimerSimulation(double y1[1])');
  time : Outport  OutDataTypeStr=double  Unit=s  PortDimensions=1  VectorParamsAs1DForOutWhenUnconnected=off
  wires:
  SFunctionDriverTimerSimulation/1 -> time/1

== system GenericTarget/Time/Task Execution Time ==
  SFunctionDriverTaskExecutionTime : S-Function  FunctionName=SFunctionDriverTaskExecutionTime  Parameters=SParameter1, SampleTime  SFunctionDeploymentMode=off  EnableBusSupport=off  mask(Legacy Function){SFunctionSpec=void OutputDriverTaskExecutionTime(double p1, double y1[1]), SParameter1=SampleTime, SampleTime=SampleTime, ShowSpec=on}
      mask prompts: SParameter1 "P1:"; SampleTime "Sample time (-1 for inherited):"; ShowSpec "Display function specification"
      mask help:
      | This block allows you to call the legacy functions specified by the following Legacy Code Tool definition:
      | def.SFunctionName = 'SFunctionDriverTaskExecutionTime';
      | def.OutputFcnSpec = 'void OutputDriverTaskExecutionTime(double p1, double y1[1])';
      | def.StartFcnSpec = 'void CreateDriverTaskExecutionTime()';
      | def.TerminateFcnSpec = 'void DeleteDriverTaskExecutionTime()';
      | def.HeaderFiles = {'DriverTaskExecutionTime.h'};
      | def.SourceFiles = {'DriverTaskExecutionTime.cpp'};
      | def.SampleTime = 'parameterized';
      | def.Options.useTlcWithAccel = false;
      mask Help: <p>This block was generated automatically by the Legacy Code Tool. For detailed help on this tool, call<a href="matlab:legacy_code('help')"> legacy_code('help')</a>.</p>
      mask Callback ShowSpec:
      | if strcmp(get_param(gcbh, 'ShowSpec'), 'on')
      |   set_param(gcbh, 'MaskDisplay', sprintf('fprintf(''%s'');', get_param(gcbh, 'SFunctionSpec')));
      | else
      |   set_param(gcbh, 'MaskDisplay', sprintf('fprintf(''%s'');', get_param(gcbh, 'FunctionName')));
      | end
      mask Display: fprintf('void OutputDriverTaskExecutionTime(double p1, double y1[1])');
  taskExecutionTime : Outport  OutDataTypeStr=double  Unit=s  PortDimensions=1  VectorParamsAs1DForOutWhenUnconnected=off
  wires:
  SFunctionDriverTaskExecutionTime/1 -> taskExecutionTime/1

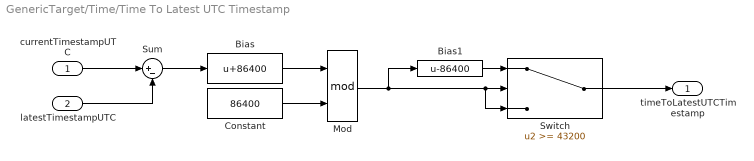
== system GenericTarget/Time/Time To Latest UTC Timestamp ==
  currentTimestampUTC : Inport  Unit=s  PortDimensions=1
  latestTimestampUTC : Inport  Port=2  Unit=s  PortDimensions=1
  Bias : Bias  Bias=86400
  Bias1 : Bias  Bias=-86400
  Constant : Constant  Value=86400
  Mod : Math  Operator=mod  SignedPower=on  SaturateOnIntegerOverflow=on
  Sum : Sum  Inputs=|+-
  Switch : Switch  Threshold=43200
  timeToLatestUTCTimestamp : Outport  Unit=s  PortDimensions=1  VectorParamsAs1DForOutWhenUnconnected=off
  wires:
  Bias1/1 -> Switch/1
  Mod/1 -> Switch/2, Switch/3, Bias1/1
  Sum/1 -> Bias/1
  Bias/1 -> Mod/1
  Switch/1 -> timeToLatestUTCTimestamp/1
  Constant/1 -> Mod/2
  currentTimestampUTC/1 -> Sum/1
  latestTimestampUTC/1 -> Sum/2

== system GenericTarget/Time/UNIX Time ==
  SFunctionDriverTimerUNIX : S-Function  FunctionName=SFunctionDriverTimerUNIX  Parameters=SampleTime  SFunctionDeploymentMode=off  EnableBusSupport=off  mask(Legacy Function){SFunctionSpec=void OutputDriverTimerUNIX(double y1[1]), SampleTime=SampleTime, ShowSpec=on}
      mask prompts: SampleTime "Sample time (-1 for inherited):"; ShowSpec "Display function specification"
      mask help:
      | This block allows you to call the legacy functions specified by the following Legacy Code Tool definition:
      | def.SFunctionName = 'SFunctionDriverTimerUNIX';
      | def.OutputFcnSpec = 'void OutputDriverTimerUNIX(double y1[1])';
      | def.StartFcnSpec = 'void CreateDriverTimerUNIX()';
      | def.TerminateFcnSpec = 'void DeleteDriverTimerUNIX()';
      | def.HeaderFiles = {'DriverTimerUNIX.h'};
      | def.SourceFiles = {'DriverTimerUNIX.cpp'};
      | def.SampleTime = 'parameterized';
      | def.Options.useTlcWithAccel = false;
      mask Help: <p>This block was generated automatically by the Legacy Code Tool. For detailed help on this tool, call<a href="matlab:legacy_code('help')"> legacy_code('help')</a>.</p>
      mask Callback ShowSpec:
      | if strcmp(get_param(gcbh, 'ShowSpec'), 'on')
      |   set_param(gcbh, 'MaskDisplay', sprintf('fprintf(''%s'');', get_param(gcbh, 'SFunctionSpec')));
      | else
      |   set_param(gcbh, 'MaskDisplay', sprintf('fprintf(''%s'');', get_param(gcbh, 'FunctionName')));
      | end
      mask Display: fprintf('void OutputDriverTimerUNIX(double y1[1])');
  time : Outport  OutDataTypeStr=double  Unit=s  PortDimensions=1  VectorParamsAs1DForOutWhenUnconnected=off
  wires:
  SFunctionDriverTimerUNIX/1 -> time/1
